simulink model "tb_MECOS_FW_v0p1"  (R2020a)
settings: Solver=ode45  StartTime=0.0  StopTime=1  MaxStep=1e-5  RelTol=1e-3
undefined symbols (not defined in the file): den_loop_filtZ, f_step, fdesignblkfcn, FPGA_CLK, FPGA_Ts, Fref, FTW_nom, G_loopfilt, gcbh, max_unwrap_periods, MECOS_A0, MECOS_A1, MECOS_A2, MECOS_B1, MECOS_B2, MECOS_cl_den, MECOS_MAX_PULSES, Nbit_Cntr, Nslits, num_loop_filtZ, PFD_noise_corrtime, PFD_Ts, phase_setpoint_degrees, PHCTRLR_CLK, PHCTRLR_Ts, Tref, unwrap_res_thr
libraries: xbsIndex_r4 x38, dspsigops x5, simulink x4, dspmlti4 x4, simulink_extras x2, dsparch4 x1, dspfdesign x1
settings Model: Creator=valbas  LastModifiedBy=valbas
settings SolverCC: AlgebraicLoopSolver=LineSearch

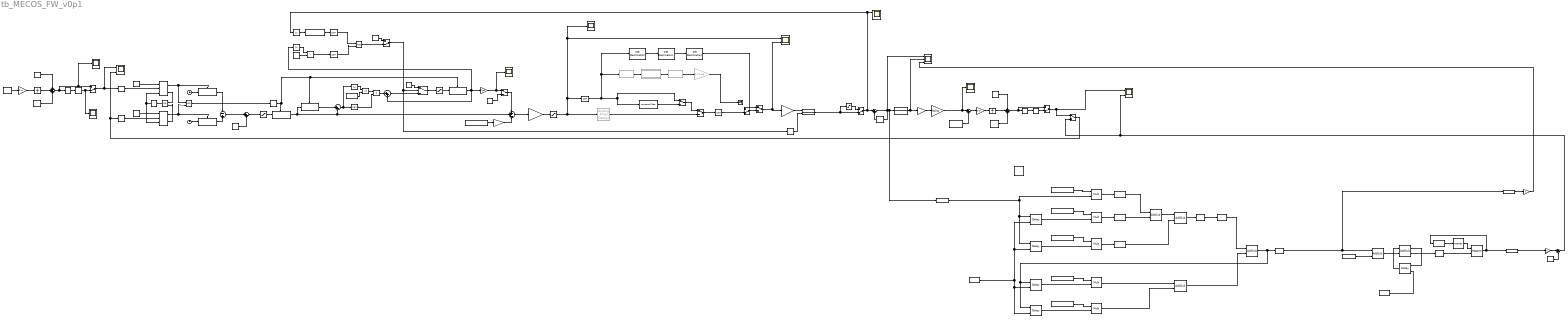
== system tb_MECOS_FW_v0p1 ==
  note: enable unwrap
  note: in a real implementation, reset downsampler filters as well
  note: if the commanded frequency variation is small
  note: unwrapper reset on frequency lock logic
  note: phase wrap detector
  note: limit phase to 0..2pi
  note: TDC
  note: AntiAlias LowPass/Averager +
      | DOWNSAMPLER
  note: Loop Filter
  note: MECOS Frequency Controller
  note: limit phase to 0..2pi
  note: PFD
  note: UNWRAPPER
  note: and we are currently unwrapping at least by one period
  note: s18_16
  note: s20_0
  note: s78_40
  note: s39_40
  note: s78_40
  note: s38_40
  note: values in green correspond to the system design on the doc;
      | sysgen does not accept more decimal places than total bits,
      | so the AnXn branch is implemented shifted by 40 positions
  note: s38_40
  note: s78_40
  note: s38_0
  note: s78_40
  note: Square-wave NCO
  note: s18_40
  note: deltaFTW command
  note: MECOS ClosedLoop IIR
  note: s78_40
  note: integral of INC/DEC steps
  note: reset
  note: s37_40
  note: s78_40
  " " : simulink/Logic and Bit Operations/Compare To Constant  relop=>=  const=0  OutDataTypeStr=boolean
  "  " : simulink/Logic and Bit Operations/Compare To Constant  relop=>=  const=0  OutDataTypeStr=boolean
  " System Generator" : xbsIndex_r4/ System Generator  Tag=genX  xilinxfamily=zynquplus  part=xczu7ev  speed=-2-e  package=ffvc1156  synthesis_tool=Vivado  clock_wrapper=Clock Enables  directory=./netlist  proj_type=Vivado  Synth_file=Vivado Synthesis Defaults  Impl_file=Vivado Implementation Defaults  testbench=off  simulink_period=FPGA_Ts  sysclk_period=FPGA_Ts*1e9  dcm_input_clock_period=10  incr_netlist=off  trim_vbits=Everywhere in SubSystem  dbl_ovrd=According to Block Masks  core_generation=According to Block Masks  run_coregen=off  deprecated_control=off  eval_field=0  block_type=sysgen
  A0 : xbsIndex_r4/Constant  const=MECOS_A0*2^40  gui_display_data_type=Fixed-point  arith_type=Signed (2's comp)  n_bits=18  bin_pt=0  preci_type=Single  exp_width=8  frac_width=24  explicit_period=off  period=1  equ=P=C  opselect=C  inp2=PCIN>>17  opr=+  inp1=P  carry=CIN  dbl_ovrd=off  block_type=constant
  A1 : xbsIndex_r4/Constant  const=MECOS_A1*2^40  gui_display_data_type=Fixed-point  arith_type=Signed (2's comp)  n_bits=18  bin_pt=0  preci_type=Single  exp_width=8  frac_width=24  explicit_period=off  period=1  equ=P=C  opselect=C  inp2=PCIN>>17  opr=+  inp1=P  carry=CIN  dbl_ovrd=off  block_type=constant
  A2 : xbsIndex_r4/Constant  const=MECOS_A2*2^40  gui_display_data_type=Fixed-point  arith_type=Signed (2's comp)  n_bits=18  bin_pt=0  preci_type=Single  exp_width=8  frac_width=24  explicit_period=off  period=1  equ=P=C  opselect=C  inp2=PCIN>>17  opr=+  inp1=P  carry=CIN  dbl_ovrd=off  block_type=constant
  Abs : Abs
  Abs1 : Abs
  Abs2 : Abs
  AddSub : xbsIndex_r4/AddSub  mode=Addition  use_carryin=off  use_carryout=on  en=off  latency=0  precision=User Defined  arith_type=Unsigned  n_bits=Nbit_Cntr  bin_pt=0  quantization=Truncate  overflow=Wrap  use_behavioral_HDL=off  hw_selection=Fabric  pipelined=off  dbl_ovrd=off  block_type=addsub
  AddSub3 : xbsIndex_r4/AddSub  mode=Addition  use_carryin=off  use_carryout=off  en=off  latency=1  precision=User Defined  arith_type=Unsigned  n_bits=Nbit_Cntr  bin_pt=0  quantization=Truncate  overflow=Saturate  use_behavioral_HDL=off  hw_selection=Fabric  pipelined=off  dbl_ovrd=off  block_type=addsub
  AddSub4 : xbsIndex_r4/AddSub  mode=Addition  use_carryin=off  use_carryout=off  en=off  latency=0  precision=Full  arith_type=Unsigned  n_bits=16  bin_pt=14  quantization=Truncate  overflow=Wrap  use_behavioral_HDL=off  hw_selection=Fabric  pipelined=off  dbl_ovrd=off  block_type=addsub
  AddSub5 : xbsIndex_r4/AddSub  mode=Addition  use_carryin=off  use_carryout=off  en=off  latency=0  precision=Full  arith_type=Unsigned  n_bits=16  bin_pt=14  quantization=Truncate  overflow=Wrap  use_behavioral_HDL=off  hw_selection=Fabric  pipelined=off  dbl_ovrd=off  block_type=addsub
  AddSub6 : xbsIndex_r4/AddSub  mode=Subtraction  use_carryin=off  use_carryout=off  en=off  latency=0  precision=User Defined  arith_type=Unsigned  n_bits=78  bin_pt=40  quantization=Truncate  overflow=Wrap  use_behavioral_HDL=off  hw_selection=Fabric  pipelined=off  dbl_ovrd=off  block_type=addsub
  AddSub7 : xbsIndex_r4/AddSub  mode=Addition  use_carryin=off  use_carryout=off  en=off  latency=0  precision=User Defined  arith_type=Unsigned  n_bits=78  bin_pt=40  quantization=Truncate  overflow=Wrap  use_behavioral_HDL=off  hw_selection=Fabric  pipelined=off  dbl_ovrd=off  block_type=addsub
  Analog Filter Design : dsparch4/Analog Filter Design  Commented=through  method=Chebyshev II  filttype=Lowpass  N=8  Wlo=100  Whi=80  Rp=2  Rs=50
  Assert : xbsIndex_r4/Assert  assert_type=on  type_source=Explicitly  gui_display_data_type=Boolean  arith_type=Boolean  n_bits=16  bin_pt=14  preci_type=Single  exp_width=8  frac_width=24  assert_rate=off  rate_source=Explicitly  period=1  output_port=on  block_type=assert
  B1 : xbsIndex_r4/Constant  const=MECOS_B1  gui_display_data_type=Fixed-point  arith_type=Signed (2's comp)  n_bits=18  bin_pt=16  preci_type=Single  exp_width=8  frac_width=24  explicit_period=off  period=1  equ=P=C  opselect=C  inp2=PCIN>>17  opr=+  inp1=P  carry=CIN  dbl_ovrd=off  block_type=constant
  B2 : xbsIndex_r4/Constant  const=MECOS_B2  gui_display_data_type=Fixed-point  arith_type=Signed (2's comp)  n_bits=18  bin_pt=16  preci_type=Single  exp_width=8  frac_width=24  explicit_period=off  period=1  equ=P=C  opselect=C  inp2=PCIN>>17  opr=+  inp1=P  carry=CIN  dbl_ovrd=off  block_type=constant
  CIC Filter : Subsystem  Commented=through  DialogController=fdesignblkfcn  InitFcn=fdesignblkfcn(gcbh, {'InitFcn'});  mask(CIC Filter){}
      mask help: Design a CIC filter
      settings: CopyFcn=fdesignblkfcn(gcbh, {'CopyFcn'});
      mask Help: helpview(mapfilelocation('dsp'), 'dspcicfilter');
      mask Display: disp('CIC')
  Clock : Clock
  Clock1 : Clock
  Command Limit : Saturate  UpperLimit=MECOS_MAX_PULSES/PHCTRLR_CLK  LowerLimit=-MECOS_MAX_PULSES/PHCTRLR_CLK
  Compare To Constant : simulink/Logic and Bit Operations/Compare To Constant  relop=<  const=unwrap_res_thr  OutDataTypeStr=boolean
  Complex to Real-Imag : ComplexToRealImag  Output=Real
  Complex to Real-Imag1 : ComplexToRealImag  Output=Real
  Constant : Constant  Value=Tref*0.9
  Constant1 : Constant  OutDataTypeStr=boolean
  Constant2 : Constant  OutDataTypeStr=boolean
  Constant3 : Constant  Value=0
  Constant4 : xbsIndex_r4/Constant  const=0  gui_display_data_type=Boolean  arith_type=Boolean  n_bits=16  bin_pt=14  preci_type=Single  exp_width=8  frac_width=24  explicit_period=off  period=1  equ=P=C  opselect=C  inp2=PCIN>>17  opr=+  inp1=P  carry=CIN  dbl_ovrd=off  block_type=constant
  Constant5 : xbsIndex_r4/Constant  const=0  gui_display_data_type=Boolean  arith_type=Boolean  n_bits=16  bin_pt=14  preci_type=Single  exp_width=8  frac_width=24  explicit_period=off  period=1  equ=P=C  opselect=C  inp2=PCIN>>17  opr=+  inp1=P  carry=CIN  dbl_ovrd=off  block_type=constant
  Constant6 : Constant  Value=0
  Constant7 : Constant  Value=0.5
  Constant8 : Constant  Value=0  OutDataTypeStr=boolean
  Constant9 : Constant
  Convert : xbsIndex_r4/Convert  gui_display_data_type=Boolean  arith_type=Boolean  n_bits=16  bin_pt=14  float_type=Single  exp_bits=8  fraction_bits=24  quantization=Truncate  overflow=Wrap  en=off  latency=1  pipeline=off  dbl_ovrd=off  block_type=convert
  Convert4 : xbsIndex_r4/Convert  gui_display_data_type=Fixed-point  arith_type="Signed  (2's comp)"  n_bits=38  bin_pt=0  float_type=Single  exp_bits=8  fraction_bits=24  quantization="Round  (unbiased: Even Values)"  overflow=Saturate  en=off  latency=1  pipeline=off  dbl_ovrd=off  block_type=convert
  Convert7 : xbsIndex_r4/Convert  gui_display_data_type=Fixed-point  arith_type="Signed  (2's comp)"  n_bits=78  bin_pt=0  float_type=Single  exp_bits=8  fraction_bits=24  quantization="Round  (unbiased: Even Values)"  overflow=Saturate  en=off  latency=0  pipeline=off  dbl_ovrd=off  block_type=convert
  D Flip-Flop : simulink_extras/Flip Flops/D Flip-Flop
  D Flip-Flop1 : simulink_extras/Flip Flops/D Flip-Flop
  Data Type Conversion : DataTypeConversion  Commented=through  OutDataTypeStr=int32  RndMeth=Round
  Data Type Conversion1 : DataTypeConversion  Commented=through  RndMeth=Round
  Delay : Delay  DelayLength=1
  Delay1 : Delay  DelayLength=1
  Delay5 : xbsIndex_r4/Delay  rst=on  infoeditControl=Selection of Reset will increase slice count due to use of real FFs and instead of SRLs  en=off  latency=2  reg_retiming=off  dbl_ovrd=off  block_type=delay
  Delay6 : xbsIndex_r4/Delay  rst=on  infoeditControl=Selection of Reset will increase slice count due to use of real FFs and instead of SRLs  en=off  latency=1  reg_retiming=off  dbl_ovrd=off  block_type=delay
  Delay7 : xbsIndex_r4/Delay  rst=on  infoeditControl=Selection of Reset will increase slice count due to use of real FFs and instead of SRLs  en=off  latency=1  reg_retiming=off  dbl_ovrd=off  block_type=delay
  Delay8 : xbsIndex_r4/Delay  rst=on  infoeditControl=Selection of Reset will increase slice count due to use of real FFs and instead of SRLs  en=off  latency=2  reg_retiming=off  dbl_ovrd=off  block_type=delay
  Delay9 : xbsIndex_r4/Delay  rst=on  infoeditControl=Selection of Reset will increase slice count due to use of real FFs and instead of SRLs  en=off  latency=1  reg_retiming=off  dbl_ovrd=off  block_type=delay
  Discrete Filter : DiscreteFilter  Numerator=num_loop_filtZ  Denominator=den_loop_filtZ  ExternalReset=Rising
      settings: InputPortMap=u0,r7
  FIR Decimation stage1 : dspmlti4/FIR Decimation  FilterSource=Dialog parameters  h=Num  D=10  filtStruct=Direct form  FilterObject=FDECIM  InputProcessing=Columns as channels (frame based)  framing=Allow multirate processing  inputOffset=0  outputBufInitCond=0  roundingMode=Floor  overflowMode=off  firstCoeffDataTypeStr=Inherit: Same word length as input  firstCoeffMin=[]  firstCoeffMax=[]  firstCoeffLastDataTypeStr=Inherit: Same word length as input  outputDataTypeStr=Inherit: Same as accumulator  outputMin=[]  outputMax=[]  outputLastDataTypeStr=Inherit: Same as accumulator
  FIR Decimation stage2 : dspmlti4/FIR Decimation  FilterSource=Dialog parameters  h=Num  D=10  filtStruct=Direct form  FilterObject=FDECIM  InputProcessing=Columns as channels (frame based)  framing=Allow multirate processing  inputOffset=0  outputBufInitCond=0  roundingMode=Floor  overflowMode=off  firstCoeffDataTypeStr=Inherit: Same word length as input  firstCoeffMin=[]  firstCoeffMax=[]  firstCoeffLastDataTypeStr=Inherit: Same word length as input  outputDataTypeStr=Inherit: Same as accumulator  outputMin=[]  outputMax=[]  outputLastDataTypeStr=Inherit: Same as accumulator
  FIR Decimation stage3 : dspmlti4/FIR Decimation  FilterSource=Dialog parameters  h=Num  D=10  filtStruct=Direct form  FilterObject=FDECIM  InputProcessing=Columns as channels (frame based)  framing=Allow multirate processing  inputOffset=0  outputBufInitCond=0  roundingMode=Floor  overflowMode=off  firstCoeffDataTypeStr=Inherit: Same word length as input  firstCoeffMin=[]  firstCoeffMax=[]  firstCoeffLastDataTypeStr=Inherit: Same word length as input  outputDataTypeStr=Inherit: Same as accumulator  outputMin=[]  outputMax=[]  outputLastDataTypeStr=Inherit: Same as accumulator
  FPGA_df : xbsIndex_r4/Gateway Out  inherit_from_input=off  hdl_port=on  rows=1  columns=1  UseAsDAC=off  DACChannel='1'  interface=None  automatic_assignment=on  address_offset=hex2dec('00')  intf_name=''  intf_description=''  timing_constraint=None  locs_specified=off  LOCs={}  io_standard={}  block_type=gatewayout
  Gain : Gain  Commented=through  Gain=1./4.e6
  Gain1 : Gain  Gain=G_loopfilt
  Gain2 : Gain  Gain=f_step
  Gain3 : Gain  Gain=2*pi
  Gain4 : Gain  Gain=FPGA_CLK
  Gain5 : Gain  Gain=2*pi
  Gain6 : Gain  Gain=Tref
  Gain7 : Gain  Gain=Tref/360
  Gain8 : Gain  Gain=2
  Gain9 : Gain
  Integrator : Integrator
  Integrator1 : Integrator
  Inverter : xbsIndex_r4/Inverter  en=off  latency=1  dbl_ovrd=off  block_type=inv
  Logical Operator : Logic  Operator=OR  IconShape=distinctive  AllPortsSameDT=off  OutDataTypeStr=boolean
  Logical Operator1 : Logic  IconShape=distinctive  AllPortsSameDT=off  OutDataTypeStr=boolean
  Logical Operator2 : Logic  Operator=XOR  IconShape=distinctive  AllPortsSameDT=off  OutDataTypeStr=boolean
  Lowpass Filter : dspfdesign/Lowpass Filter  FilterType=FIR  DesignForMinimumOrder=on  FilterOrder=50  PassbandFrequency=30  StopbandFrequency=70  PassbandRipple=1  StopbandAttenuation=30  InheritSampleRate=off  SampleRate=100e3  SimulateUsing=Interpreted execution  roundingMode=Floor  coeffsDataTypeStr=fixdt(1,16)
  MECOS Df Hz : Scope
  MECOS closed loop : TransferFcn  Denominator=MECOS_cl_den
  MECOS cmd pulses : Scope  NumInputPorts=3
  MECOS_OUT : xbsIndex_r4/Gateway Out  inherit_from_input=off  hdl_port=on  rows=1  columns=1  UseAsDAC=off  DACChannel='1'  interface=None  automatic_assignment=on  address_offset=hex2dec('00')  intf_name=''  intf_description=''  timing_constraint=None  locs_specified=off  LOCs={}  io_standard={}  block_type=gatewayout
  MECOS_df : Scope  NumInputPorts=3
  Magnitude-Angle to Complex : MagnitudeAngleToComplex  Input=Angle  ConstantPart=1
  Magnitude-Angle to Complex1 : MagnitudeAngleToComplex  Input=Angle  ConstantPart=1
  Manual Switch{,1,4..5} (4 alike) : ManualSwitch  CurrentSetting=0
  Manual Switch{2..3,6..8} (5 alike) : ManualSwitch
  Memory : Memory
  Memory1 : Memory
  Mult1 : xbsIndex_r4/Mult  precision=Full  arith_type="Signed  (2's comp)"  n_bits=16  bin_pt=14  quantization=Truncate  overflow=Wrap  en=off  latency=0  use_behavioral_HDL=off  opt=Speed  use_embedded=on  optimum_pipeline=off  pipeline=on  dbl_ovrd=off  use_rpm=on  placement_style=Triangular  block_type=mult
  Mult2 : xbsIndex_r4/Mult  precision=Full  arith_type="Signed  (2's comp)"  n_bits=16  bin_pt=14  quantization=Truncate  overflow=Wrap  en=off  latency=0  use_behavioral_HDL=off  opt=Speed  use_embedded=on  optimum_pipeline=off  pipeline=on  dbl_ovrd=off  use_rpm=on  placement_style=Triangular  block_type=mult
  Mult3 : xbsIndex_r4/Mult  precision=User Defined  arith_type="Signed  (2's comp)"  n_bits=78  bin_pt=40  quantization=Truncate  overflow=Wrap  en=off  latency=0  use_behavioral_HDL=off  opt=Speed  use_embedded=on  optimum_pipeline=off  pipeline=on  dbl_ovrd=off  use_rpm=on  placement_style=Triangular  block_type=mult
  Mult4 : xbsIndex_r4/Mult  precision=Full  arith_type="Signed  (2's comp)"  n_bits=16  bin_pt=14  quantization=Truncate  overflow=Wrap  en=off  latency=0  use_behavioral_HDL=off  opt=Speed  use_embedded=on  optimum_pipeline=off  pipeline=on  dbl_ovrd=off  use_rpm=on  placement_style=Triangular  block_type=mult
  Mult5 : xbsIndex_r4/Mult  precision=User Defined  arith_type="Signed  (2's comp)"  n_bits=78  bin_pt=40  quantization=Truncate  overflow=Wrap  en=off  latency=0  use_behavioral_HDL=off  opt=Speed  use_embedded=on  optimum_pipeline=off  pipeline=on  dbl_ovrd=off  use_rpm=on  placement_style=Triangular  block_type=mult
  Nominal_VCO_FTW : xbsIndex_r4/Constant  const=FTW_nom  gui_display_data_type=Fixed-point  arith_type=Signed (2's comp)  n_bits=Nbit_Cntr+1  bin_pt=0  preci_type=Single  exp_width=8  frac_width=24  explicit_period=on  period=FPGA_Ts  equ=P=C  opselect=C  inp2=PCIN>>17  opr=+  inp1=P  carry=CIN  dbl_ovrd=off  block_type=constant
  Not necessary but just to be safe : Saturate  UpperLimit=Tref  LowerLimit=-Tref
  Product : Product
  Ref freq : Constant  Value=Fref+1
  Ref initial phase (rad) : Constant  Value=0
  Ref ph noise : Constant  Value=0
  Register : xbsIndex_r4/Register  init=0  rst=off  en=on  dbl_ovrd=off  block_type=register
  Reinterpret : xbsIndex_r4/Reinterpret  force_arith_type=off  arith_type=Unsigned  force_bin_pt=on  bin_pt=40  block_type=reinterpret
  Relational Operator : RelationalOperator  OutDataTypeStr=boolean  RndMeth=Simplest
  Relational Operator1 : RelationalOperator  Operator=>  OutDataTypeStr=boolean  RndMeth=Simplest
  Sample Ref Edge : dspsigops/Sample and Hold  trig=Rising edge  initCond=0  latchinput=on
  Sample VCO Edge : dspsigops/Sample and Hold  trig=Rising edge  initCond=0  latchinput=on
  Slice : xbsIndex_r4/Slice  nbits=37  boolean_output=off  mode=Upper Bit Location + Width  bit1=-1  base1=MSB of Input  bit0=0  base0=LSB of Input  dbl_ovrd=off  block_type=slice
  Slice1 : xbsIndex_r4/Slice  nbits=37  boolean_output=off  mode=Upper Bit Location + Width  bit1=-1  base1=MSB of Input  bit0=0  base0=LSB of Input  dbl_ovrd=off  block_type=slice
  Slice2 : xbsIndex_r4/Slice  nbits=37  boolean_output=off  mode=Upper Bit Location + Width  bit1=-1  base1=MSB of Input  bit0=0  base0=LSB of Input  dbl_ovrd=off  block_type=slice
  Sum{,1,6,8} (4 alike) : Sum  Inputs=|++
  Sum2 : Sum  Inputs=+++
  Sum3 : Sum  Inputs=+++
  Sum4 : Sum  Inputs=-|+
  Sum5 : Sum  Inputs=|+-
  Sum7 : Sum  Inputs=++-
  Sum9 : Sum  Inputs=|+-
  Switch : Switch  Criteria=u2 > Threshold
  Terminator : Terminator
  Time pulse : dspsigops/Sample and Hold  trig=Falling edge  initCond=0  latchinput=on
  VCO : Scope  NumInputPorts=2
  VCO initial phase (rad) : Constant  Value=0
  VCO ph noise : Constant  Value=0
  VCO quiescent freq : Constant  Value=Fref
  Zero-Order Hold1 : ZeroOrderHold  SampleTime=PHCTRLR_Ts
  Zero-Order Hold2 : ZeroOrderHold  SampleTime=PFD_Ts
  Zero-Order Hold3 : ZeroOrderHold  SampleTime=PHCTRLR_Ts
  Zero-Order Hold4 : ZeroOrderHold  SampleTime=PHCTRLR_Ts
  corr_sign : Signum
  decim_TDC : Scope  NumInputPorts=2
  enable unwrap reset : ManualSwitch  CurrentSetting=0
  max correction : Saturate  UpperLimit=max_unwrap_periods  LowerLimit=-max_unwrap_periods
  max correction1 : Saturate  UpperLimit=max_unwrap_periods*Tref*FPGA_CLK  LowerLimit=-max_unwrap_periods*Tref*FPGA_CLK
  not_decim_TDC : Scope
  num periods to unwrap : dspsigops/Sample and Hold  trig=Falling edge  initCond=0  latchinput=on
  ph_setpoint : Constant  Value=phase_setpoint_degrees
  prev time pulse : dspsigops/Sample and Hold  trig=Falling edge  initCond=0  latchinput=on
  signals : Scope  NumInputPorts=2
  slits : Gain  Gain=Nslits
  t_correction : Scope
  time jitter : simulink/Sources/Band-Limited White Noise  Cov=PFD_jitter_PSD  Ts=PFD_noise_corrtime  seed=[23341]
  tot_steps : xbsIndex_r4/Gateway In  gui_display_data_type=Fixed-point  arith_type="Signed  (2's comp)"  n_bits=20  bin_pt=0  preci_type=Single  exp_width=8  frac_width=24  rows=1  columns=1  quantization="Round  (unbiased: +/- Inf)"  overflow=Saturate  period=MECOS_Ts  UseAsADC=off  ADCChannel='1'  interface=None  automatic_assignment=on  address_offset=hex2dec('00')  intf_name=''  intf_description=''  default_value=0  timing_constraint=None  locs_specified=off  LOCs={}  io_standard={}  inherit_from_input=off  hdl_port=on  dbl_ovrd=off  block_type=gatewayin
  unwrapped : Scope
  wrapped : Scope
  wires:
  Gain1/1 -> Discrete Filter/1
  Manual Switch6/1 -> decim_TDC/2, Gain1/1  "decim TDC out"
  Delay1/1 -> Sum/2
  Sum/1 -> Delay1/1, tot_steps/1, MECOS closed loop/1, MECOS_df/1
  MECOS closed loop/1 -> Gain2/1, MECOS_df/2
  slits/1 -> MECOS Df Hz/1, Sum1/1  "deltaf"
  VCO quiescent freq/1 -> Sum1/2
  Sum1/1 -> Gain3/1
  Gain3/1 -> Integrator/1  "w"
  Integrator/1 -> Sum3/2  "ph"
  Magnitude-Angle to Complex/1 -> Complex to Real-Imag1/1
  Magnitude-Angle to Complex1/1 -> Complex to Real-Imag/1
  Gain5/1 -> Integrator1/1
  Ref freq/1 -> Gain5/1
  VCO initial phase (rad)/1 -> Sum3/3
  Sum3/1 -> Manual Switch1/1, Magnitude-Angle to Complex/1
  Sum2/1 -> unwrapped/1, Manual Switch/1, Magnitude-Angle to Complex1/1
  Complex to Real-Imag/1 -> wrapped/1, Manual Switch/2
  max correction1/1 -> not_decim_TDC/1, decim_TDC/1, Zero-Order Hold2/1, Analog Filter Design/1  "not decim TDC out"
  Manual Switch/1 -> signals/1, " "/1
  Complex to Real-Imag1/1 -> Manual Switch1/2
  Discrete Filter/1 -> Command Limit/1, Manual Switch4/2
  Lowpass Filter/1 -> Manual Switch7/2
  Analog Filter Design/1 -> Manual Switch2/2
  Manual Switch2/1 -> Zero-Order Hold1/1
  " "/1 -> D Flip-Flop/2
  Sample Ref Edge/1 -> Sum4/1
  "  "/1 -> D Flip-Flop1/2
  Manual Switch8/1 -> "  "/1, signals/2
  Sample VCO Edge/1 -> Sum4/2
  Clock/1 -> Sample Ref Edge/1
  Clock1/1 -> Sample VCO Edge/1
  Sum4/1 -> Sum8/1
  Logical Operator2/1 -> Memory/1
  Logical Operator/1 -> Memory1/1
  D Flip-Flop1/2 -> Logical Operator/2
  Constant2/1 -> D Flip-Flop1/1
  Memory1/1 -> D Flip-Flop1/3, D Flip-Flop/3
  D Flip-Flop/2 -> Logical Operator/1
  Constant1/1 -> D Flip-Flop/1
  D Flip-Flop/1 -> Logical Operator2/1, Sample Ref Edge/Trigger  "UP"
  D Flip-Flop1/1 -> Logical Operator2/2, Sample VCO Edge/Trigger  "DOWN"
  Sum5/1 -> Abs/1, corr_sign/1
  Constant/1 -> Relational Operator/2
  Abs/1 -> Relational Operator/1
  num periods to unwrap/1 -> Sum6/2, Abs2/1, Gain6/1
  corr_sign/1 -> Product/2
  Sum6/1 -> Switch/3
  Gain6/1 -> t_correction/1, Manual Switch3/1
  Constant3/1 -> Manual Switch3/2
  Manual Switch3/1 -> Sum7/1
  prev time pulse/1 -> Sum5/1
  Time pulse/1 -> prev time pulse/1, Sum5/2, Sum7/2
  Command Limit/1 -> Manual Switch4/1
  Not necessary but just to be safe/1 -> Time pulse/1
  Data Type Conversion/1 -> CIC Filter/1(In)
  CIC Filter/1(Out) -> Data Type Conversion1/1
  Data Type Conversion1/1 -> Gain/1
  Zero-Order Hold1/1 -> Manual Switch5/2
  Gain/1 -> Terminator/1
  Manual Switch5/1 -> Manual Switch6/2  "decim TDC out"
  FIR Decimation stage1/1 -> FIR Decimation stage2/1
  FIR Decimation stage2/1 -> FIR Decimation stage3/1
  FIR Decimation stage3/1 -> Manual Switch6/1
  Integrator1/1 -> Sum2/2
  Ref initial phase (rad)/1 -> Sum2/3
  VCO ph noise/1 -> Sum3/1
  Manual Switch7/1 -> Manual Switch2/1
  Zero-Order Hold2/1 -> FIR Decimation stage1/1, Data Type Conversion/1, Manual Switch7/1, Lowpass Filter/1
  max correction/1 -> num periods to unwrap/1
  Sum7/1 -> Gain4/1
  Gain4/1 -> max correction1/1  "not decim TDC out"
  Ref ph noise/1 -> Sum2/1
  Switch/1 -> max correction/1
  Abs1/1 -> Compare To Constant/1
  Compare To Constant/1 -> Zero-Order Hold3/1
  Relational Operator/1 -> Product/1
  Product/1 -> Sum6/1
  Memory/1 -> Time pulse/Trigger, num periods to unwrap/Trigger, prev time pulse/Trigger
  Delay/1 -> Discrete Filter/2
  Constant7/1 -> Relational Operator1/2
  Relational Operator1/1 -> Zero-Order Hold4/1
  enable unwrap reset/1 -> Delay/1, Switch/2  "filt_reset"
  Manual Switch4/1 -> Abs1/1, MECOS cmd pulses/1, Sum/1
  Zero-Order Hold4/1 -> Logical Operator1/2
  Abs2/1 -> Relational Operator1/1
  Zero-Order Hold3/1 -> Logical Operator1/1
  Constant8/1 -> enable unwrap reset/1
  ph_setpoint/1 -> Gain7/1
  Gain7/1 -> Sum7/3
  Constant6/1 -> Switch/1
  Logical Operator1/1 -> enable unwrap reset/2  "filt_reset"
  Sum8/1 -> Not necessary but just to be safe/1
  time jitter/1 -> Sum8/2
  Gain2/1 -> slits/1  "deltaf"
  A1/1 -> Mult2/1
  Slice/1 -> AddSub5/1
  Mult1/1 -> Slice/1
  Delay6/1 -> Mult2/2
  Mult2/1 -> Slice1/1
  AddSub7/1 -> AddSub6/2
  Convert4/1 -> FPGA_df/1, AddSub3/1
  A2/1 -> Mult4/1
  AddSub5/1 -> AddSub4/1
  Delay7/1 -> Mult3/2
  Constant4/1 -> Delay6/2, Delay5/2, Delay8/2, Delay7/2
  Mult5/1 -> AddSub7/2
  B2/1 -> Mult5/1
  Mult4/1 -> Slice2/1
  Nominal_VCO_FTW/1 -> AddSub3/2
  AddSub3/1 -> AddSub/2
  Slice1/1 -> AddSub5/2
  A0/1 -> Mult1/1
  AddSub/1 -> Delay9/1
  Assert/1 -> Inverter/1
  AddSub6/1 -> Delay7/1, Delay8/1, Convert4/1
  AddSub/2 -> Convert/1
  Mult3/1 -> AddSub7/1
  Register/1 -> Assert/1, MECOS_OUT/1
  Delay5/1 -> Mult4/2
  Inverter/1 -> Register/1
  Convert/1 -> Register/2
  Delay8/1 -> Mult5/2
  Slice2/1 -> AddSub4/2
  B1/1 -> Mult3/1
  AddSub4/1 -> Convert7/1
  Reinterpret/1 -> AddSub6/1
  Delay9/1 -> AddSub/1
  Convert7/1 -> Reinterpret/1
  tot_steps/1 -> Delay6/1, Delay5/1, Mult1/2
  Constant5/1 -> Delay9/2
  MECOS_OUT/1 -> Gain8/1
  Gain8/1 -> Sum9/1
  Constant9/1 -> Sum9/2
  Sum9/1 -> Manual Switch8/2, VCO/2
  Manual Switch1/1 -> Manual Switch8/1, VCO/1
  FPGA_df/1 -> Gain9/1
  Gain9/1 -> MECOS_df/3

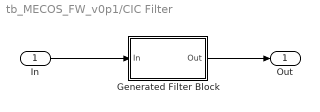
== system tb_MECOS_FW_v0p1/CIC Filter ==
  In : Inport
  Generated Filter Block : Subsystem  Tag=BlockMethodSubSystem
  Out : Outport  VectorParamsAs1DForOutWhenUnconnected=off
  wires:
  In/1 -> Generated Filter Block/1(In)
  Generated Filter Block/1(Out) -> Out/1

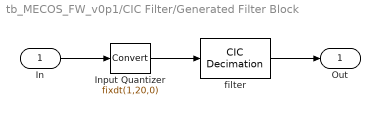
== system tb_MECOS_FW_v0p1/CIC Filter/Generated Filter Block ==
  In : Inport
  Input Quantizer : DataTypeConversion  OutDataTypeStr=fixdt(1,20,0)  RndMeth=Round  SaturateOnIntegerOverflow=on
  filter : dspmlti4/CIC Decimation  filtFrom=Dialog parameters  filtobj=CICDECIM  ftype=Decimator  R=1000  M=2  N=2  filterInternals=Full precision  BPS=[42 42 42 42]  FLPS=[0 0 0 0]  outputWordLength=42  outputFracLength=0  launchFVT=off  framing=Maintain input frame rate  RateOptions=Allow multirate processing
      settings: SourceProductBaseCode=DS
  Out : Outport
  wires:
  In/1 -> Input Quantizer/1
  Input Quantizer/1 -> filter/1
  filter/1 -> Out/1
